simulink model "test_filter"  (R2022a)
settings: Solver=VariableStepAuto  StartTime=0.0  StopTime=3  RelTol=1e-3
undefined symbols (not defined in the file or in its folder): generator
settings Model: Creator=Niccolò  LastModifiedBy=Niccolò

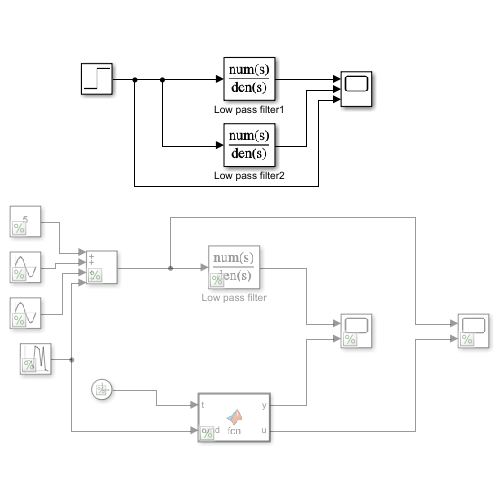
[thumbnail: Simulink's stored preview of the top-level diagram]
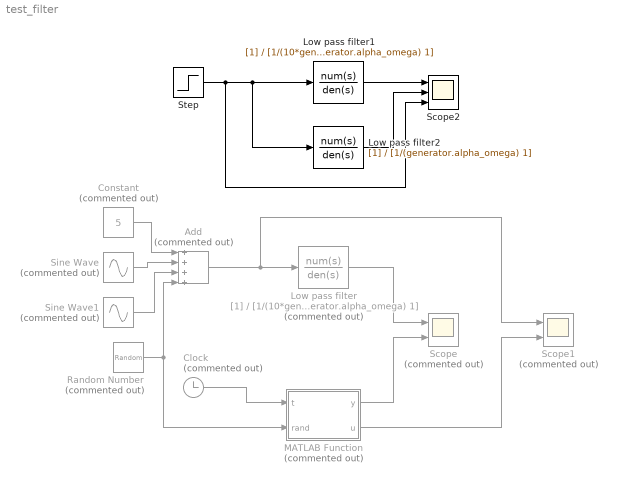
== system test_filter ==
  Add : Sum  Commented=on  Inputs=++++
  Clock : Clock  Commented=on
  Constant : Constant  Commented=on  Value=5
  Low pass filter : TransferFcn  Commented=on  Denominator=[1/(10*generator.alpha_omega) 1]
  Low pass filter1 : TransferFcn  Denominator=[1/(10*generator.alpha_omega) 1]
  Low pass filter2 : TransferFcn  Denominator=[1/(generator.alpha_omega) 1]
  MATLAB Function : MATLAB Function  Commented=on  TreatAsAtomicUnit=on
  Random Number : RandomNumber  Commented=on  SampleTime=0.1
  Scope : Scope  Commented=on  NumInputPorts=2
  Scope1 : Scope  Commented=on  NumInputPorts=2
  Scope2 : Scope  NumInputPorts=3
  Sine Wave : Sin  Commented=on  Amplitude=0.3  Frequency=1e4  SampleTime=0
  Sine Wave1 : Sin  Commented=on  Amplitude=10  Frequency=1e-1  SampleTime=0
  Step : Step  SampleTime=0
  wires:
  Sine Wave/1 -> Add/2
  Sine Wave1/1 -> Add/3
  Add/1 -> Scope1/1, Low pass filter/1
  Low pass filter/1 -> Scope/1
  MATLAB Function/1(y) -> Scope/2
  MATLAB Function/2(u) -> Scope1/2
  Constant/1 -> Add/1
  Clock/1 -> MATLAB Function/1(t)
  Random Number/1 -> MATLAB Function/2(rand), Add/4
  Low pass filter1/1 -> Scope2/1
  Step/1 -> Scope2/3, Low pass filter2/1, Low pass filter1/1
  Low pass filter2/1 -> Scope2/2

== matlab function test_filter/MATLAB Function ==
  data: y output; t input; u output; generator parameter; rand input
function [y, u] = fcn(t, generator, rand)
u = 0.3*sin(1e4*t) + 10*sin(0.1*t) + rand +5;
% windowSize = 5; 
% b = (1/windowSize)*ones(1,windowSize);
% a = 1;
b = 1;
a = [generator.alpha_omega 1];
y = filter(b, a, u);
